simulink model "Air_Controller"  (R2017a)
settings: Solver=ode45  StartTime=0.0  StopTime=600  RelTol=1e-3
undefined symbols (not defined in the file): sigbuilder_block
settings Model: Creator=Mohanad M.Marzouk  LastModifiedBy=Mohanad M.Marzouk
settings DebuggingCC: SignalRangeChecking=error

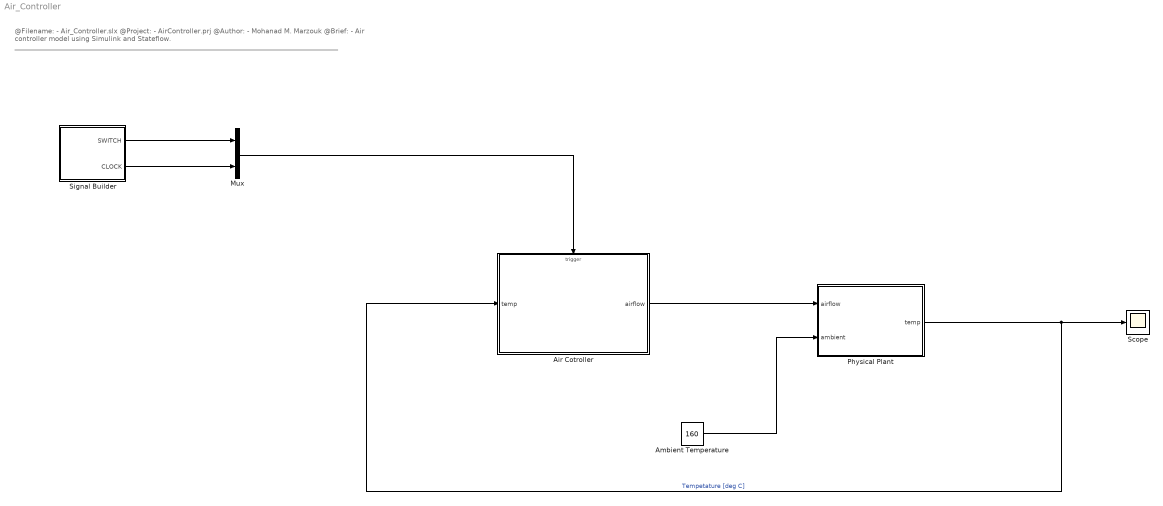
== system Air_Controller ==
  note: @Filename: - Air_Controller.slx
      | @Project: - AirController.prj
      | @Author: - Mohanad M. Marzouk
      | @Brief: - Air controller model using Simulink and Stateflow.
      | _________________________________________________________________________________________________
  Air Cotroller : Stateflow chart  TreatAsAtomicUnit=on
  Ambient Temperature : Constant  Value=160
  Mux : Mux  Inputs=2
  Physical Plant : Subsystem
  Scope : Scope
  Signal Builder : Subsystem  Tag=STV Subsys  LoadFcn=sigbuilder_block('load');  StartFcn=sigbuilder_block('start');  StopFcn=sigbuilder_block('stop');  ClipboardFcn=sigbuilder_block('clipboard');  mask(Sigbuilder block){tuvar=[0:10]}
      mask help: Simulink:masks:SigbuilderBlock_MD
      mask init:
      | if ~strcmp(get_param(bdroot(gcbh),'SimulationStatus'),'stopped') tuvar = sigbuilder_block('maskInit'); end
      settings: CopyFcn=sigbuilder_block('copy');  DeleteFcn=sigbuilder_block('delete');  ModelCloseFcn=sigbuilder_block('modelClose');  PreSaveFcn=sigbuilder_block('preSave');  PauseFcn=sigbuilder_block('pause');  ContinueFcn=sigbuilder_block('continue');  NameChangeFcn=sigbuilder_block('namechange');  OpenFcn=sigbuilder_block('open',[0 30 1024.5 488.25 ]);  CloseFcn=sigbuilder_block('close');
      mask Display: plot(0, 0, 100, 100,[2, 2, 32, 32, 2], [68, 8, 8, 68, 68],[32, 2], [38, 38], [32, 19, 2],[53, 60, 44], [32, 17, 17, 2],[16, 16, 31, 31]);txt = getActiveGroup(gcbh);text(2, 100, txt,'verticalAlignment', 'top');
  wires:
  Signal Builder/1(SWITCH) -> Mux/1
  Signal Builder/2(CLOCK) -> Mux/2
  Physical Plant/1(temp) -> Air Cotroller/1(temp), Scope/1  "Tempetature [deg C]"
  Ambient Temperature/1 -> Physical Plant/2(ambient)
  Air Cotroller/1(airflow) -> Physical Plant/1(airflow)
  Mux/1 -> Air Cotroller/Trigger

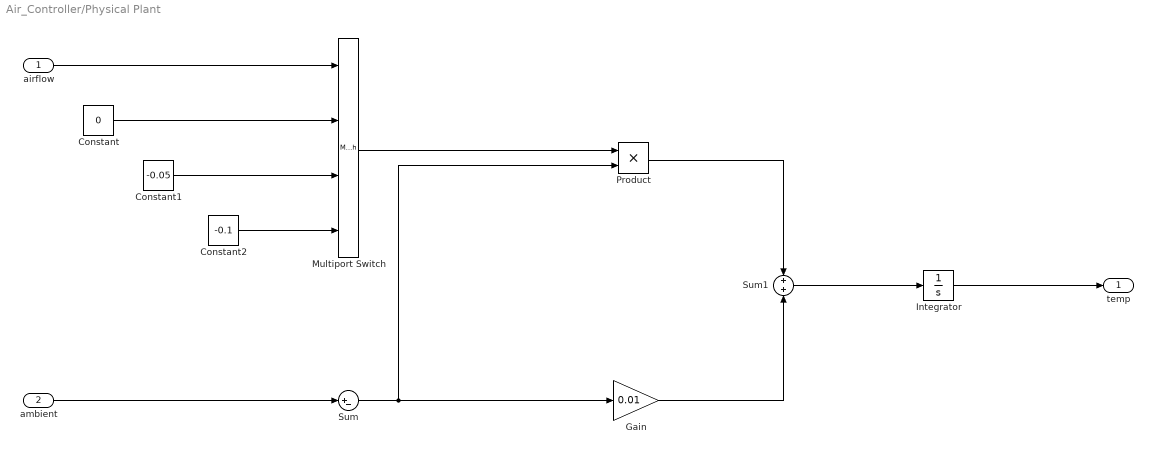
== system Air_Controller/Physical Plant ==
  airflow : Inport
  ambient : Inport  Port=2
  Constant : Constant  Value=0
  Constant1 : Constant  Value=-0.05
  Constant2 : Constant  Value=-0.1
  Gain : Gain  Gain=0.01
  Integrator : Integrator  InitialCondition=70
  Multiport Switch : MultiPortSwitch  DataPortOrder=Zero-based contiguous
  Product : Product
  Sum : Sum  Inputs=|+-
  Sum1 : Sum  Inputs=+|+
  temp : Outport
  wires:
  Constant2/1 -> Multiport Switch/4
  Constant1/1 -> Multiport Switch/3
  Constant/1 -> Multiport Switch/2
  airflow/1 -> Multiport Switch/1
  Multiport Switch/1 -> Product/1
  ambient/1 -> Sum/1
  Sum/1 -> Product/2, Gain/1
  Product/1 -> Sum1/1
  Gain/1 -> Sum1/2
  Sum1/1 -> Integrator/1
  Integrator/1 -> temp/1

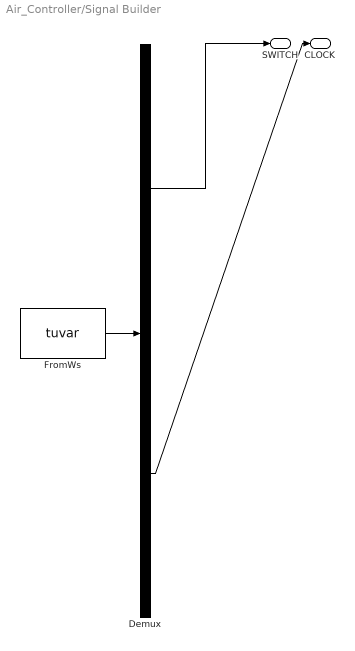
== system Air_Controller/Signal Builder ==
  Demux : Demux  Tag=STV Demux  Outputs=2
  FromWs : FromWorkspace  Tag=STV FromWs  VariableName=tuvar  SampleTime=0
      SigBuilderData=|
      | common.afterFinalStr = 'Extrapolate'
      | common.sampleTime = 0
      | dataSet.timeRange = [0 600]
      | dataSet.name = 'Group 1'
      | sbobj.Groups.Name = 'Group 1'
      | sbobj.Groups.Signals(1).Name = 'SWITCH'
      | sbobj.Groups.Signals(1).XData = [0 350 350 501 501 600]
      | sbobj.Groups.Signals(1).YData = [0 0 1 1 0 0]
      | sbobj.Groups.Signals(2).Name = 'CLOCK'
      | sbobj.Groups.Signals(2).XData = [0 0 0.5 0.5 1 1 1.5 1.5 2 2 2.5 2.5 ... (2402 elements, 1x2402)]
      | sbobj.Groups.Signals(2).YData = [0 2 2 0 0 2 2 0 0 2 2 0 ... (2402 elements, 1x2402)]
      | sbobj.Groups.TimeRange = [0 600]
  SWITCH : Outport  Tag=STV Outport
  CLOCK : Outport  Tag=STV Outport  Port=2
  wires:
  Demux/1 -> SWITCH/1
  FromWs/1 -> Demux/1
  Demux/2 -> CLOCK/1

== stateflow chart Air_Controller/Air Cotroller ==
  settings: executeAtInitialization=1
  state PowerOn
    state FAN1 [parallel]
      settings: executionOrder=1
      state On
      state Off
      PowerOn.FAN1.On -> PowerOn.FAN1.Off : [temp < 120]
      (default) -> PowerOn.FAN1.Off
      PowerOn.FAN1.Off -> PowerOn.FAN1.On : [temp >= 120]
    state FAN2 [parallel]
      settings: executionOrder=2
      state On
      state Off
      PowerOn.FAN2.On -> PowerOn.FAN2.Off : [temp < 150]
      (default) -> PowerOn.FAN2.Off
      PowerOn.FAN2.Off -> PowerOn.FAN2.On : [temp >= 150]
    state SpeedValue [parallel]
      during: airflow = in(FAN1.On) + in(FAN2.On);
      settings: executionOrder=3
  state PowerOff
    entry: airflow = 0;
  PowerOff -> PowerOn : SWITCH
  PowerOn -> PowerOff : SWITCH
  (default) -> PowerOff
  data: temp input; airflow output uint8 [0..2]
  events: SWITCH input EITHER_EDGE_EVENT; CLOCK input EITHER_EDGE_EVENT
